simulink model "InvertedPendulumSimOpenLoopTemplate"  (Simulink 9.2)
settings: Solver=ode5  StartTime=0.0  StopTime=3  FixedStep=0.01  RelTol=1e-3
PreLoadFcn:
  | InvertedPendulumSimOpenLoopSolutionInit
InitFcn:
  | clear PlotPendulum
undefined symbols (not defined in the file): fc, fp, Fs, g, J, l, m, M, mp, OffsetPend, PlotPendulum, sigmaCart, sigmaPend, Ts, x0
libraries: simulink x4
settings Model: Creator=jims  LastModifiedBy=root  ExtModeTrigDuration=12000  ExtModeTrigLevel=0.400000
settings DataIOCC: LimitDataPoints=off  SignalLoggingSaveFormat=Dataset  SaveOutput=off  SignalLogging=off  DSMLogging=off  SaveTime=off  SignalLoggingName=sigsOut
settings OptimizationCC: EfficientFloat2IntCast=on  SimCompilerOptimization=on
settings DebuggingCC: SaveWithParameterizedLinksMsg=none  UnderspecifiedInitializationDetection=Simplified  MergeDetectMultiDrivingBlocksExec=error  IntegerOverflowMsg=none  FcnCallInpInsideContextMsg=error  UniqueDataStoreMsg=error  AssertControl=DisableAll  StateNameClashWarn=none  StrictBusMsg=ErrorOnBusTreatedAsVector  IntegerSaturationMsg=none
settings HardwareCC: ProdIntDivRoundTo=Zero  ProdEndianess=LittleEndian  ProdHWDeviceType=Intel->x86/Pentium
settings SFSimCC: SimParseCustomCode=off
settings RTWCC: SystemTargetFile=rtwin.tlc  TemplateMakefile=rtwin.tmf  Description=Real-Time Windows Target  RTWCompilerOptimization=on
settings TargetCC: TargetLibSuffix=_rtwin.lib  TargetPreCompLibLocation=C:\Program Files\MATLAB\R2014a\toolbox\rtw\targets\rtwin\lib\win64  PreserveStateflowLocalDataDimensions=off
settings CustomProperty: DataType=string

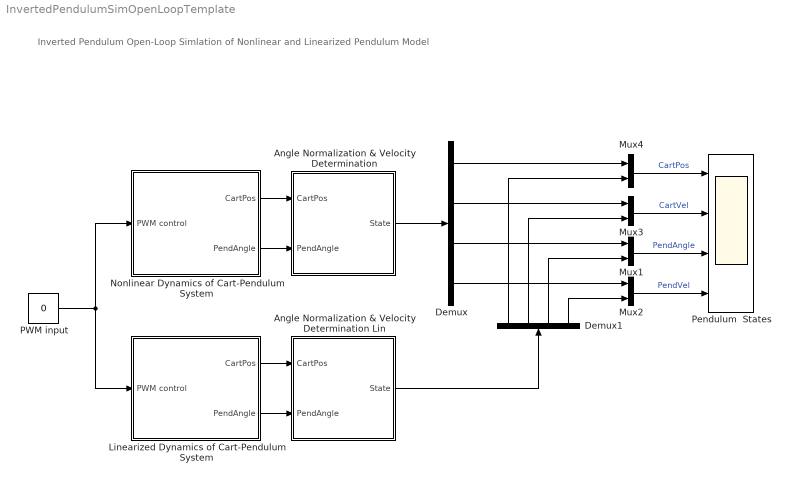
== system InvertedPendulumSimOpenLoopTemplate ==
  note: Inverted Pendulum Open-Loop Simlation of
      | Nonlinear and Linearized Pendulum Model
  Angle Normalization & Velocity Determination : Subsystem
  Angle Normalization & Velocity Determination Lin : Subsystem
  Demux : Demux
  Demux1 : Demux
  Linearized Dynamics of Cart-Pendulum System : Subsystem  mask(Simulation of Pendulum Dynamics){}
      mask Display:
      | plot( [0.725 0.725], [1.15 0.375]); % pendulum arm
      | plot(0.725+0.05*sin([0:0.5:7]), 0.325+0.05*cos([0:0.5:7])); % pendulum load mass
      | plot([-0.2], [-0.2]);
      | plot([1.9], [1.7]);
      | plot([0.1 1.4], [1.09 1.09]); % upper rail
      | plot([0.1 1.4], [1.07 1.07]); % upper rail
      | plot([0.65 0.8], [1.1 1.1]); % cart bottom
      | plot([0.65 0.8], [1.2 1.2]); % cart top
      | plot([0.65 0.65], [1.2 1.1]); % cart left
      | plot([0.8 0.8], [1.1 1.2]); % cart right
      | port_label('input', 1, 'PWM');
      | port_label('output', 1, 'CartPos');
      | port_label('output', 2, 'PendAngle');
  Mux{1..4} (4 alike) : Mux  Inputs=2
  Nonlinear Dynamics of Cart-Pendulum System : Subsystem  mask(Simulation of Pendulum Dynamics){}
      mask Display:
      | plot( [0.725 0.725], [1.15 0.375]); % pendulum arm
      | plot(0.725+0.05*sin([0:0.5:7]), 0.325+0.05*cos([0:0.5:7])); % pendulum load mass
      | plot([-0.2], [-0.2]);
      | plot([1.9], [1.7]);
      | plot([0.1 1.4], [1.09 1.09]); % upper rail
      | plot([0.1 1.4], [1.07 1.07]); % upper rail
      | plot([0.65 0.8], [1.1 1.1]); % cart bottom
      | plot([0.65 0.8], [1.2 1.2]); % cart top
      | plot([0.65 0.65], [1.2 1.1]); % cart left
      | plot([0.8 0.8], [1.1 1.2]); % cart right
      | port_label('input', 1, 'PWM');
      | port_label('output', 1, 'CartPos');
      | port_label('output', 2, 'PendAngle');
  PWM input : Constant  Value=0
  Pendulum  States : Scope  NumInputPorts=4
  wires:
  Mux4/1 -> Pendulum  States/1  "CartPos"
  Mux3/1 -> Pendulum  States/2  "CartVel"
  Demux/4 -> Mux2/1
  Demux/3 -> Mux1/1
  Demux/2 -> Mux3/1
  Demux/1 -> Mux4/1
  Angle Normalization & Velocity Determination/1(State) -> Demux/1
  Demux1/1 -> Mux4/2
  Demux1/2 -> Mux3/2
  Demux1/3 -> Mux1/2
  Demux1/4 -> Mux2/2
  Mux1/1 -> Pendulum  States/3  "PendAngle"
  Mux2/1 -> Pendulum  States/4  "PendVel"
  Nonlinear Dynamics of Cart-Pendulum System/1(CartPos) -> Angle Normalization & Velocity Determination/1(CartPos)
  Nonlinear Dynamics of Cart-Pendulum System/2(PendAngle) -> Angle Normalization & Velocity Determination/2(PendAngle)
  Linearized Dynamics of Cart-Pendulum System/1(CartPos) -> Angle Normalization & Velocity Determination Lin/1(CartPos)
  Linearized Dynamics of Cart-Pendulum System/2(PendAngle) -> Angle Normalization & Velocity Determination Lin/2(PendAngle)
  Angle Normalization & Velocity Determination Lin/1(State) -> Demux1/1
  PWM input/1 -> Nonlinear Dynamics of Cart-Pendulum System/1(PWM control), Linearized Dynamics of Cart-Pendulum System/1(PWM control)

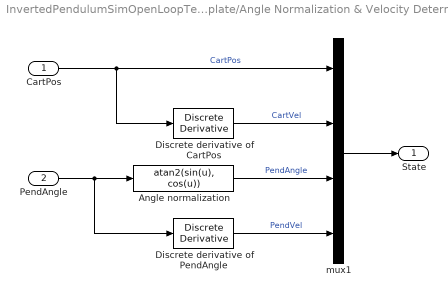
== system InvertedPendulumSimOpenLoopTemplate/Angle Normalization & Velocity Determination ==
  CartPos : Inport
  PendAngle : Inport  Port=2
  Angle normalization : Fcn  Expr=atan2(sin(u), cos(u))
  Discrete derivative of CartPos : simulink/Discrete/Discrete Derivative  gainval=1.0  ICPrevScaledInput=x0(1)/Ts  OutMin=[]  OutMax=[]  OutDataType=sfix(16)  OutScaling=2^-10  DoSatur=off
  Discrete derivative of PendAngle : simulink/Discrete/Discrete Derivative  gainval=1.0  ICPrevScaledInput=x0(3)/Ts  OutMin=[]  OutMax=[]  OutDataType=sfix(16)  OutScaling=2^-10  DoSatur=off
  mux1 : Mux
  State : Outport
  wires:
  Discrete derivative of PendAngle/1 -> mux1/4  "PendVel"
  Angle normalization/1 -> mux1/3  "PendAngle"
  Discrete derivative of CartPos/1 -> mux1/2  "CartVel"
  PendAngle/1 -> Discrete derivative of PendAngle/1, Angle normalization/1
  mux1/1 -> State/1
  CartPos/1 -> mux1/1, Discrete derivative of CartPos/1  "CartPos"

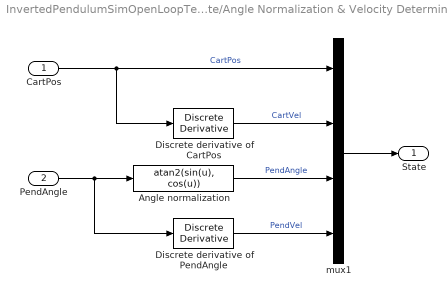
== system InvertedPendulumSimOpenLoopTemplate/Angle Normalization & Velocity Determination Lin ==
  CartPos : Inport
  PendAngle : Inport  Port=2
  Angle normalization : Fcn  Expr=atan2(sin(u), cos(u))
  Discrete derivative of CartPos : simulink/Discrete/Discrete Derivative  gainval=1.0  ICPrevScaledInput=x0(1)/Ts  OutMin=[]  OutMax=[]  OutDataType=sfix(16)  OutScaling=2^-10  DoSatur=off
  Discrete derivative of PendAngle : simulink/Discrete/Discrete Derivative  gainval=1.0  ICPrevScaledInput=x0(3)/Ts  OutMin=[]  OutMax=[]  OutDataType=sfix(16)  OutScaling=2^-10  DoSatur=off
  mux1 : Mux
  State : Outport
  wires:
  Discrete derivative of PendAngle/1 -> mux1/4  "PendVel"
  Angle normalization/1 -> mux1/3  "PendAngle"
  Discrete derivative of CartPos/1 -> mux1/2  "CartVel"
  PendAngle/1 -> Discrete derivative of PendAngle/1, Angle normalization/1
  mux1/1 -> State/1
  CartPos/1 -> mux1/1, Discrete derivative of CartPos/1  "CartPos"

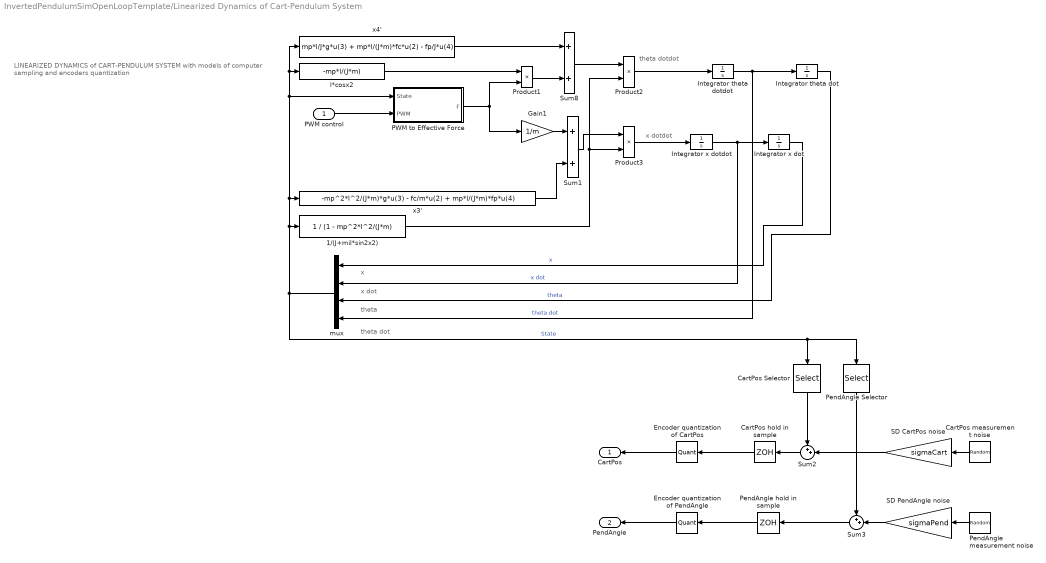
== system InvertedPendulumSimOpenLoopTemplate/Linearized Dynamics of Cart-Pendulum System ==
  note: x
  note: x dot
  note: theta
  note: theta dot
  note: x dotdot
  note: theta dotdot
  note: LINEARIZED DYNAMICS of CART-PENDULUM SYSTEM
      | with models of computer sampling and encoders quantization
  PWM control : Inport
  1/(J+mil*sin2x2) : Fcn  Expr=1 / (1 - mp^2*l^2/(J*m)
  CartPos hold in sample : ZeroOrderHold  SampleTime=Ts
  CartPos measurement noise : RandomNumber  SampleTime=Ts
  CartPos Selector : Selector  InputPortWidth=4  IndexOptions=Index vector (dialog)  Indices=[1]  OutputSizes=1
  Encoder quantization of CartPos : Quantizer  QuantizationInterval=ResCartEnc
  Encoder quantization of PendAngle : Quantizer  QuantizationInterval=ResPendEnc
  Gain1 : Gain  Gain=1/m  SaturateOnIntegerOverflow=on  OutDataTypeStr=Inherit: Same as input  ParamDataTypeStr=Inherit: Same as input
  Integrator theta dot : Integrator  InitialCondition=x0(3)
  Integrator theta dotdot : Integrator  InitialCondition=x0(4)
  Integrator x dot : Integrator  InitialCondition=x0(1)
  Integrator x dotdot : Integrator  InitialCondition=x0(2)
  PWM to Effective Force : Subsystem
  PendAngle hold in sample : ZeroOrderHold  SampleTime=Ts
  PendAngle measurement noise : RandomNumber  SampleTime=Ts
  PendAngle Selector : Selector  InputPortWidth=4  IndexOptions=Index vector (dialog)  Indices=[3]  OutputSizes=1
  Product1 : Product  SaturateOnIntegerOverflow=on  InputSameDT=on  OutDataTypeStr=Inherit: Same as first input
  Product2 : Product  SaturateOnIntegerOverflow=on  InputSameDT=on  OutDataTypeStr=Inherit: Same as first input
  Product3 : Product  SaturateOnIntegerOverflow=on  InputSameDT=on  OutDataTypeStr=Inherit: Same as first input
  SD CartPos noise : Gain  Gain=sigmaCart  SaturateOnIntegerOverflow=on  OutDataTypeStr=Inherit: Same as input  ParamDataTypeStr=Inherit: Same as input
  SD PendAngle noise : Gain  Gain=sigmaPend  SaturateOnIntegerOverflow=on  OutDataTypeStr=Inherit: Same as input  ParamDataTypeStr=Inherit: Same as input
  Sum1 : Sum  SaturateOnIntegerOverflow=on  InputSameDT=on  OutDataTypeStr=Inherit: Same as first input
  Sum2 : Sum  Inputs=++|  SaturateOnIntegerOverflow=on  InputSameDT=on  OutDataTypeStr=Inherit: Same as first input
  Sum3 : Sum  Inputs=++|  SaturateOnIntegerOverflow=on  InputSameDT=on  OutDataTypeStr=Inherit: Same as first input
  Sum8 : Sum  SaturateOnIntegerOverflow=on  InputSameDT=on  OutDataTypeStr=Inherit: Same as first input
  l*cosx2 : Fcn  Expr=-mp*l/(J*m)
  mux : Mux
  x3' : Fcn  Expr=-mp^2*l^2/(J*m)*g*u(3) - fc/m*u(2) + mp*l/(J*m)*fp*u(4)
  x4' : Fcn  Expr=mp*l/J*g*u(3) + mp*l/(J*m)*fc*u(2) - fp/J*u(4)
  CartPos : Outport
  PendAngle : Outport  Port=2
  wires:
  PWM control/1 -> PWM to Effective Force/2(PWM)
  mux/1 -> CartPos Selector/1, PendAngle Selector/1, PWM to Effective Force/1(State), x4'/1, l*cosx2/1, x3'/1, 1/(J+mil*sin2x2)/1  "State"
  CartPos hold in sample/1 -> Encoder quantization of CartPos/1
  Encoder quantization of CartPos/1 -> CartPos/1
  PendAngle hold in sample/1 -> Encoder quantization of PendAngle/1
  Encoder quantization of PendAngle/1 -> PendAngle/1
  Sum2/1 -> CartPos hold in sample/1
  SD CartPos noise/1 -> Sum2/2
  CartPos measurement noise/1 -> SD CartPos noise/1
  Sum3/1 -> PendAngle hold in sample/1
  SD PendAngle noise/1 -> Sum3/2
  PendAngle measurement noise/1 -> SD PendAngle noise/1
  CartPos Selector/1 -> Sum2/1
  PendAngle Selector/1 -> Sum3/1
  PWM to Effective Force/1(F) -> Gain1/1, Product1/2
  l*cosx2/1 -> Product1/1
  Product1/1 -> Sum8/2
  x4'/1 -> Sum8/1
  Sum8/1 -> Product2/1
  1/(J+mil*sin2x2)/1 -> Product3/2, Product2/2
  Product2/1 -> Integrator theta dotdot/1
  Gain1/1 -> Sum1/1
  x3'/1 -> Sum1/2
  Sum1/1 -> Product3/1
  Product3/1 -> Integrator x dotdot/1
  Integrator theta dotdot/1 -> Integrator theta dot/1, mux/4  "theta dot"
  Integrator x dotdot/1 -> Integrator x dot/1, mux/2  "x dot"
  Integrator theta dot/1 -> mux/3  "theta"
  Integrator x dot/1 -> mux/1  "x"

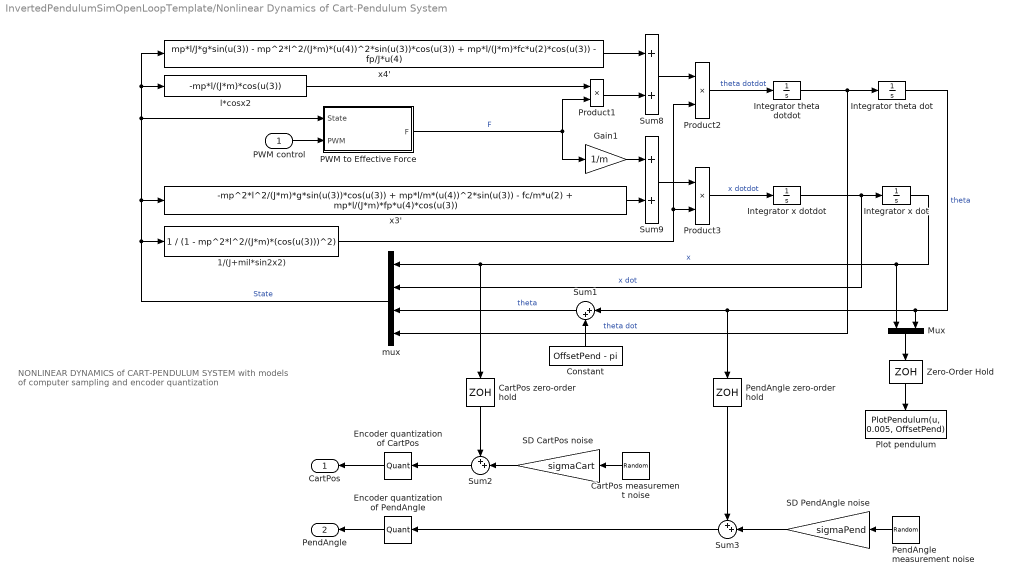
== system InvertedPendulumSimOpenLoopTemplate/Nonlinear Dynamics of Cart-Pendulum System ==
  note: NONLINEAR DYNAMICS of CART-PENDULUM
      | SYSTEM with models of computer sampling
      | and encoder quantization
  PWM control : Inport
  1/(J+mil*sin2x2) : Fcn  Expr=1 / (1 - mp^2*l^2/(J*m)*(cos(u(3)))^2)
  CartPos measurement noise : RandomNumber  SampleTime=Ts
  CartPos zero-order hold : ZeroOrderHold  SampleTime=Ts
  Constant : Constant  Value=OffsetPend - pi
  Encoder quantization of CartPos : Quantizer  QuantizationInterval=ResCartEnc
  Encoder quantization of PendAngle : Quantizer  QuantizationInterval=ResPendEnc
  Gain1 : Gain  Gain=1/m  SaturateOnIntegerOverflow=on  OutDataTypeStr=Inherit: Same as input  ParamDataTypeStr=Inherit: Same as input
  Integrator theta dot : Integrator  InitialCondition=x0(3)
  Integrator theta dotdot : Integrator  InitialCondition=x0(4)
  Integrator x dot : Integrator  InitialCondition=x0(1)
  Integrator x dotdot : Integrator  InitialCondition=x0(2)
  Mux : Mux  Inputs=2
  PWM to Effective Force : Subsystem
  PendAngle measurement noise : RandomNumber  SampleTime=Ts
  PendAngle zero-order hold : ZeroOrderHold  SampleTime=Ts
  Plot pendulum : MATLABFcn  MATLABFcn=PlotPendulum(u, 0.005, OffsetPend)  OutputDimensions=0
  Product1 : Product  SaturateOnIntegerOverflow=on  InputSameDT=on  OutDataTypeStr=Inherit: Same as first input
  Product2 : Product  SaturateOnIntegerOverflow=on  InputSameDT=on  OutDataTypeStr=Inherit: Same as first input
  Product3 : Product  SaturateOnIntegerOverflow=on  InputSameDT=on  OutDataTypeStr=Inherit: Same as first input
  SD CartPos noise : Gain  Gain=sigmaCart  SaturateOnIntegerOverflow=on  OutDataTypeStr=Inherit: Same as input  ParamDataTypeStr=Inherit: Same as input
  SD PendAngle noise : Gain  Gain=sigmaPend  SaturateOnIntegerOverflow=on  OutDataTypeStr=Inherit: Same as input  ParamDataTypeStr=Inherit: Same as input
  Sum1 : Sum  Inputs=|++  SaturateOnIntegerOverflow=on  InputSameDT=on  OutDataTypeStr=Inherit: Same as first input
  Sum2 : Sum  Inputs=++|  SaturateOnIntegerOverflow=on  InputSameDT=on  OutDataTypeStr=Inherit: Same as first input
  Sum3 : Sum  Inputs=++|  SaturateOnIntegerOverflow=on  InputSameDT=on  OutDataTypeStr=Inherit: Same as first input
  Sum8 : Sum  SaturateOnIntegerOverflow=on  InputSameDT=on  OutDataTypeStr=Inherit: Same as first input
  Sum9 : Sum  SaturateOnIntegerOverflow=on  InputSameDT=on  OutDataTypeStr=Inherit: Same as first input
  Zero-Order Hold : ZeroOrderHold  SampleTime=Ts
  l*cosx2 : Fcn  Expr=-mp*l/(J*m)*cos(u(3))
  mux : Mux
  x3' : Fcn  Expr=-mp^2*l^2/(J*m)*g*sin(u(3))*cos(u(3)) + mp*l/m*(u(4))^2*sin(u(3)) - fc/m*u(2) + mp*l/(J*m)*fp*u(4)*cos(u(3))
  x4' : Fcn  Expr=mp*l/J*g*sin(u(3)) - mp^2*l^2/(J*m)*(u(4))^2*sin(u(3))*cos(u(3)) + mp*l/(J*m)*fc*u(2)*cos(u(3)) - fp/J*u(4)
  CartPos : Outport
  PendAngle : Outport  Port=2
  wires:
  Sum2/1 -> Encoder quantization of CartPos/1
  mux/1 -> 1/(J+mil*sin2x2)/1, x3'/1, l*cosx2/1, x4'/1, PWM to Effective Force/1(State)  "State"
  Encoder quantization of CartPos/1 -> CartPos/1
  Integrator theta dotdot/1 -> mux/4, Integrator theta dot/1  "theta dot"
  l*cosx2/1 -> Product1/1
  Product1/1 -> Sum8/2
  Product2/1 -> Integrator theta dotdot/1  "theta dotdot"
  Product3/1 -> Integrator x dotdot/1  "x dotdot"
  Sum9/1 -> Product3/1
  Integrator x dotdot/1 -> Integrator x dot/1, mux/2  "x dot"
  PWM to Effective Force/1(F) -> Product1/2, Gain1/1  "F"
  x3'/1 -> Sum9/2
  Gain1/1 -> Sum9/1
  Sum8/1 -> Product2/1
  x4'/1 -> Sum8/1
  1/(J+mil*sin2x2)/1 -> Product2/2, Product3/2
  PWM control/1 -> PWM to Effective Force/2(PWM)
  Sum3/1 -> Encoder quantization of PendAngle/1
  SD CartPos noise/1 -> Sum2/2
  CartPos measurement noise/1 -> SD CartPos noise/1
  SD PendAngle noise/1 -> Sum3/2
  PendAngle measurement noise/1 -> SD PendAngle noise/1
  Integrator theta dot/1 -> Mux/2, Sum1/1, PendAngle zero-order hold/1  "theta"
  Integrator x dot/1 -> Mux/1, mux/1, CartPos zero-order hold/1  "x"
  Sum1/1 -> mux/3  "theta"
  Constant/1 -> Sum1/2
  Mux/1 -> Zero-Order Hold/1
  Zero-Order Hold/1 -> Plot pendulum/1
  CartPos zero-order hold/1 -> Sum2/1
  PendAngle zero-order hold/1 -> Sum3/1
  Encoder quantization of PendAngle/1 -> PendAngle/1

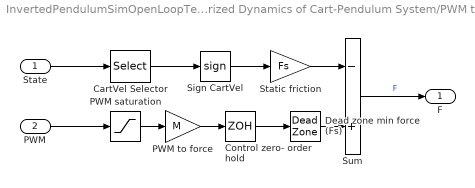
== system InvertedPendulumSimOpenLoopTemplate/Linearized Dynamics of Cart-Pendulum System/PWM to Effective Force ==
  State : Inport
  PWM : Inport  Port=2
  CartVel Selector : Selector  InputPortWidth=4  IndexOptions=Index vector (dialog)  Indices=[2]  OutputSizes=1
  Control zero- order hold : ZeroOrderHold  SampleTime=Ts
  Dead zone min force (Fs) : DeadZone  LowerValue=-Fs  UpperValue=Fs  SaturateOnIntegerOverflow=on
  PWM saturation : Saturate
  PWM to force : Gain  Gain=M  SaturateOnIntegerOverflow=on  OutDataTypeStr=Inherit: Same as input  ParamDataTypeStr=Inherit: Same as input
  Sign CartVel : Signum
  Static friction : Gain  Gain=Fs  SaturateOnIntegerOverflow=on  OutDataTypeStr=Inherit: Same as input  ParamDataTypeStr=Inherit: Same as input
  Sum : Sum  Inputs=-+  SaturateOnIntegerOverflow=on  InputSameDT=on  OutDataTypeStr=Inherit: Same as first input
  F : Outport
  wires:
  State/1 -> CartVel Selector/1
  Static friction/1 -> Sum/1
  PWM to force/1 -> Control zero- order hold/1
  Control zero- order hold/1 -> Dead zone min force (Fs)/1
  Dead zone min force (Fs)/1 -> Sum/2
  Sign CartVel/1 -> Static friction/1
  PWM saturation/1 -> PWM to force/1
  Sum/1 -> F/1  "F"
  PWM/1 -> PWM saturation/1
  CartVel Selector/1 -> Sign CartVel/1

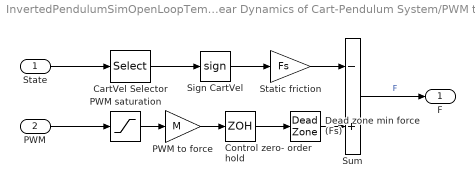
== system InvertedPendulumSimOpenLoopTemplate/Nonlinear Dynamics of Cart-Pendulum System/PWM to Effective Force ==
  State : Inport
  PWM : Inport  Port=2
  CartVel Selector : Selector  InputPortWidth=4  IndexOptions=Index vector (dialog)  Indices=[2]  OutputSizes=1
  Control zero- order hold : ZeroOrderHold  SampleTime=Ts
  Dead zone min force (Fs) : DeadZone  LowerValue=-Fs  UpperValue=Fs  SaturateOnIntegerOverflow=on
  PWM saturation : Saturate
  PWM to force : Gain  Gain=M  SaturateOnIntegerOverflow=on  OutDataTypeStr=Inherit: Same as input  ParamDataTypeStr=Inherit: Same as input
  Sign CartVel : Signum
  Static friction : Gain  Gain=Fs  SaturateOnIntegerOverflow=on  OutDataTypeStr=Inherit: Same as input  ParamDataTypeStr=Inherit: Same as input
  Sum : Sum  Inputs=-+  SaturateOnIntegerOverflow=on  InputSameDT=on  OutDataTypeStr=Inherit: Same as first input
  F : Outport
  wires:
  State/1 -> CartVel Selector/1
  Static friction/1 -> Sum/1
  PWM to force/1 -> Control zero- order hold/1
  Control zero- order hold/1 -> Dead zone min force (Fs)/1
  Dead zone min force (Fs)/1 -> Sum/2
  Sign CartVel/1 -> Static friction/1
  PWM saturation/1 -> PWM to force/1
  Sum/1 -> F/1  "F"
  PWM/1 -> PWM saturation/1
  CartVel Selector/1 -> Sign CartVel/1
